simulink model "model"  (R2020a)
settings: Solver=VariableStepAuto  StartTime=0.0  StopTime=4  RelTol=1e-3
values from neighbouring files (symbols this model uses):
  a = a(pav)    [fcn_u.m]    (also in parametry.m)
  b = b(pav)    [fcn_u.m]    (also in parametry.m)
  c = c(pav)    [fcn_u.m]    (also in parametry.m)
  d = d(pav)    [fcn_u.m]    (also in parametry.m)
  g = 9.81    [parametry.m]
  Jw = 0.01    [parametry.m]
  mw = 1200    [parametry.m]
  rw = 0.30    (= 0.3)    [parametry.m]
  Tb = 300    [parametry.m]
  Vpocz = 20    [parametry.m]
settings Model: Creator=lukas  LastModifiedBy=lukas
settings SolverCC: ZeroCrossControl=EnableAll  ZeroCrossAlgorithm=Adaptive
settings DebuggingCC: IgnoredZcDiagnostic=none
settings HardwareCC: ProdHWDeviceType=AMD->x86-64 (Windows64)

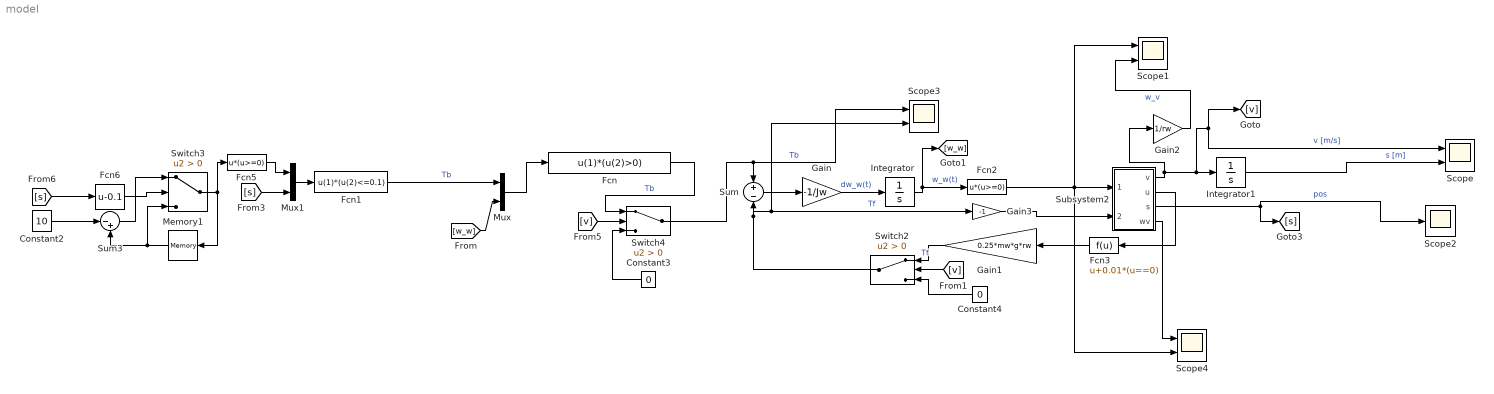
== system model ==
  Constant2 : Constant  Value=10
  Constant3 : Constant  Value=0
  Constant4 : Constant  Value=0
  Fcn : Fcn  Expr=u(1)*(u(2)>0)
  Fcn1 : Fcn  Expr=u(1)*(u(2)<=0.1)
  Fcn2 : Fcn  Expr=u*(u>=0)
  Fcn3 : Fcn  Expr=u+0.01*(u==0)
  Fcn5 : Fcn  Expr=u*(u>=0)
  Fcn6 : Fcn  Expr=u-0.1
  Gain : Gain  Gain=-1/Jw
  Gain1 : Gain  Gain=0.25*mw*g*rw
  Gain2 : Gain  Gain=1/rw
  Gain3 : Gain  Gain=-1
  Integrator : Integrator  InitialCondition=Vpocz/rw
  Integrator1 : Integrator
  Memory1 : Memory  InitialCondition=Tb
  Mux : Mux  Inputs=2
  Mux1 : Mux  Inputs=2
  Scope{,1,3..4} (4 alike) : Scope  NumInputPorts=2
  Scope2 : Scope
  Subsystem2 : Subsystem
  Sum : Sum  Inputs=+-
  Sum3 : Sum  Inputs=|-+
  Switch2 : Switch  Criteria=u2 > Threshold
  Switch3 : Switch  Criteria=u2 > Threshold
  Switch4 : Switch  Criteria=u2 > Threshold
  wires:
  Gain/1 -> Integrator/1  "dw_w(t)"
  Subsystem2/2(u) -> Fcn3/1
  Subsystem2/1(v) -> Gain2/1, Scope/1, [v], Integrator1/1  "v [m/s]"
  Integrator1/1 -> Scope/2  "s [m]"
  Sum/1 -> Gain/1
  Gain1/1 -> Switch2/1  "Tf"
  Constant4/1 -> Switch2/3
  Fcn1/1 -> Mux/1  "Tb"
  [v] -> Switch2/2
  [w_w] -> Mux/2
  Subsystem2/3(s) -> Scope2/1, [s]  "pos"
  Mux/1 -> Fcn/1
  Gain2/1 -> Scope1/2  "w_v"
  Integrator/1 -> Fcn2/1, [w_w]  "w_w(t)"
  Subsystem2/4(wv) -> Scope4/1
  Gain3/1 -> Subsystem2/2(-Ff*rw)
  Switch2/1 -> Scope3/2, Gain3/1, Sum/2  "Tf"
  Mux1/1 -> Fcn1/1
  [s] -> Mux1/2
  Fcn2/1 -> Scope4/2, Scope1/1, Subsystem2/1(w_w(t))
  Fcn3/1 -> Gain1/1
  Fcn5/1 -> Mux1/1
  Memory1/1 -> Switch3/3, Sum3/2
  Constant2/1 -> Sum3/1
  Switch3/1 -> Fcn5/1, Memory1/1
  [s] -> Fcn6/1
  Fcn6/1 -> Switch3/2
  [v] -> Switch4/2
  Switch4/1 -> Scope3/1, Sum/1  "Tb"
  Constant3/1 -> Switch4/3
  Fcn/1 -> Switch4/1  "Tb"
  Sum3/1 -> Switch3/1

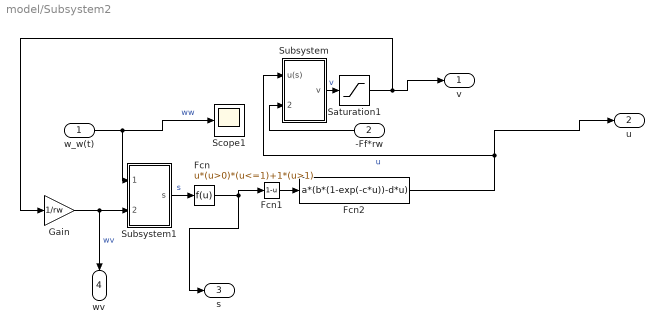
== system model/Subsystem2 ==
  w_w(t) : Inport
  -Ff*rw : Inport  Port=2
  Fcn : Fcn  Expr=u*(u>0)*(u<=1)+1*(u>1)
  Fcn1 : Fcn  Expr=1-u
  Fcn2 : Fcn  Expr=a*(b*(1-exp(-c*u))-d*u)
  Gain : Gain  Gain=1/rw
  Saturation1 : Saturate  UpperLimit=inf  LowerLimit=0
  Scope1 : Scope
  Subsystem : Subsystem
  Subsystem1 : Subsystem
  v : Outport
  u : Outport  Port=2
  s : Outport  Port=3
  wv : Outport  Port=4
  wires:
  w_w(t)/1 -> Scope1/1, Subsystem1/1(w_w(t))  "ww"
  Gain/1 -> Subsystem1/2(w_v(t)), wv/1  "wv"
  Subsystem/1(v) -> Saturation1/1  "v"
  Saturation1/1 -> Gain/1, v/1
  Subsystem1/1(s) -> Fcn/1  "s"
  Fcn/1 -> Fcn1/1, s/1
  Fcn1/1 -> Fcn2/1
  Fcn2/1 -> u/1, Subsystem/1(u(s))  "u"
  -Ff*rw/1 -> Subsystem/2(-Ff*rw)

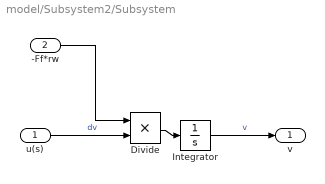
== system model/Subsystem2/Subsystem ==
  u(s) : Inport
  -Ff*rw : Inport  Port=2
  Divide : Product  Inputs=**
  Integrator : Integrator  InitialCondition=Vpocz
  v : Outport
  wires:
  u(s)/1 -> Divide/2  "dv"
  Integrator/1 -> v/1  "v"
  Divide/1 -> Integrator/1
  -Ff*rw/1 -> Divide/1

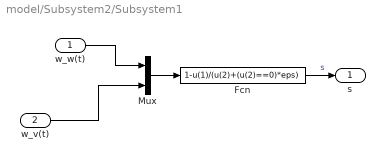
== system model/Subsystem2/Subsystem1 ==
  w_w(t) : Inport
  w_v(t) : Inport  Port=2
  Fcn : Fcn  Expr=1-u(1)/(u(2)+(u(2)==0)*eps)
  Mux : Mux  Inputs=2
  s : Outport
  wires:
  Fcn/1 -> s/1  "s"
  w_v(t)/1 -> Mux/2
  Mux/1 -> Fcn/1
  w_w(t)/1 -> Mux/1
